simulink model "verify_entropy_mdl"  (R2013b)
settings: Solver=FixedStepDiscrete  StartTime=0.0  StopTime=1  FixedStep=1  RelTol=1e-3
values from neighbouring files (symbols this model uses):
  fmix = mix(n)    [verification_density.m]    (also in verification_fluidproperty.m; verification_heat_capacity.m; verification_kinematic_viscosity.m; verification_thermal_conductivity.m)
  press = p(m)    [verification_density.m]    (also in verification_fluidproperty.m; verification_heat_capacity.m; verification_kinematic_viscosity.m; verification_thermal_conductivity.m)
undefined symbols (not defined in the file or in its folder): fluid
libraries: carnot x1
settings Model: Creator=drhf  LastModifiedBy=drhf
settings DataIOCC: SignalLoggingSaveFormat=ModelDataLogs  SaveTime=off  ReturnWorkspaceOutputs=on  OutputSaveName=rho2
settings OptimizationCC: ExpressionDepthLimit=2147483647
settings DebuggingCC: FcnCallInpInsideContextMsg=UseLocalSettings  FrameProcessingCompatibilityMsg=error  StateNameClashWarn=warning
settings GRTTargetCC: CodeReplacementLibrary=C89/C90 (ANSI)  CombineOutputUpdateFcns=off  GRTInterface=on

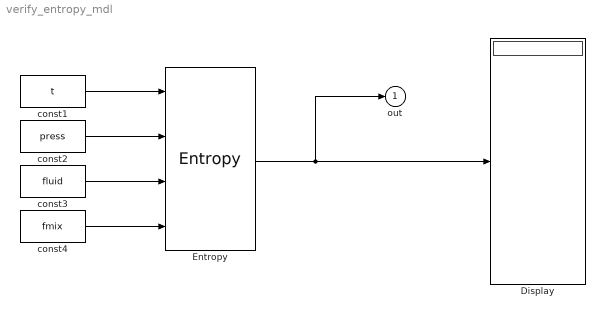
== system verify_entropy_mdl ==
  Display : Display
  Entropy : carnot/Basic/Material_Properties/Entropy  VariantControl=CarlibClassic  INPUTARGUMENTS=state variables (classic)  DEBUGLEVEL=NOLEVEL  MAXTOTALMESSAGES=inf  MAXCONSECUTIVEMESSAGES=inf  WRITETOFILE=0  FILENAME='errors.txt'
  const1 : Constant  Value=t
  const2 : Constant  Value=press
  const3 : Constant  Value=fluid
  const4 : Constant  Value=fmix
  out : Outport  InitialOutput=0
  wires:
  Entropy/1 -> Display/1, out/1
  const1/1 -> Entropy/1
  const2/1 -> Entropy/2
  const3/1 -> Entropy/3
  const4/1 -> Entropy/4
